simulink model "comboPlusKirschBinarized"  (R2024a)
settings: Solver=FixedStepDiscrete  StartTime=0.0  StopTime=1  RelTol=1e-3
undefined symbols (not defined in the file or in its folder): dx, dy, G, KirschThrL, KirschThrS, MagThr, north, northWest, southWest, west
libraries: visionsinks x10, hdlsllib x8, visionsources x1
Description:
  | Sobel Edge Detection Using the MATLAB(R) Function Block
  | This example shows how to use HDL Coder(TM) to check,
  | generate, and verify HDL code for a Sobel Edge Detection
  | block built using the MATLAB Function block.
settings Model: FPTRunName=Active  Creator=The MathWorks, Inc.  LastModifiedBy=dskap
settings SolverCC: AlgebraicLoopSolver=TrustRegion
settings DataIOCC: LimitDataPoints=on  SaveFormat=Array  SignalLogging=off  ReturnWorkspaceOutputs=off
settings OptimizationCC: BlockReduction=off  ConditionallyExecuteInputs=off  DefaultParameterBehavior=Inlined  ExpressionDepthLimit=2147483647  InitFltsAndDblsToZero=on  EfficientMapNaN2IntZero=off  LifeSpan=inf
settings DebuggingCC: AlgebraicLoopMsg=error  SaveWithParameterizedLinksMsg=none  UnderspecifiedInitializationDetection=Classic  MergeDetectMultiDrivingBlocksExec=none  SignalResolutionControl=TryResolveAllWithWarning  MultiTaskDSMMsg=warning  MultiTaskCondExecSysMsg=none  SingleTaskRateTransMsg=error  IntegerOverflowMsg=none  ParameterPrecisionLossMsg=none  FcnCallInpInsideContextMsg=warning  UnconnectedInputMsg=warning  UnconnectedOutputMsg=warning  UnconnectedLineMsg=warning  AllowSymbolicDim=off  StateNameClashWarn=warning  StrictBusMsg=ErrorOnBusTreatedAsVector  SFUnexpectedBacktrackingDiag=warning  SFNoUnconditionalDefaultTransitionDiag=warning  SFExecutionAtInitializationDiag=none  IntegerSaturationMsg=none  ArithmeticOperatorsInVariantConditions=warning
settings HardwareCC: ProdBitPerPointer=32  ProdBitPerSizeT=32  ProdBitPerPtrDiffT=32  ProdLargestAtomicFloat=None  ProdIntDivRoundTo=Undefined  ProdEndianess=Unspecified  ProdWordSize=32  ProdHWDeviceType=ASIC/FPGA  TargetHWDeviceType=32-bit Generic  ProdEqTarget=off
settings ModelReferenceCC: EnableRefExpFcnMdlSchedulingChecks=on  PropagateSignalLabelsOutOfModel=off
settings SFSimCC: SimUseLocalCustomCode=off  CustomCodeUndefinedFunction=UseInterfaceOnly
settings RTWCC: RTWUseLocalCustomCode=off  GPUComputeCapability=3.5  DLArmComputeVersion=19.05
settings CodeAppCC: StateflowObjectComments=on
settings GRTTargetCC: TargetFcnLib=ansi_tfl_tmw.mat  TargetLangStandard=C89/C90 (ANSI)  CombineOutputUpdateFcns=off  GRTInterface=on
settings ConfigComp: CovMetricSettings=dw  CovSaveCumulativeToWorkspaceVar=on  CovSaveSingleToWorkspaceVar=on  CovExternalEMLEnable=off

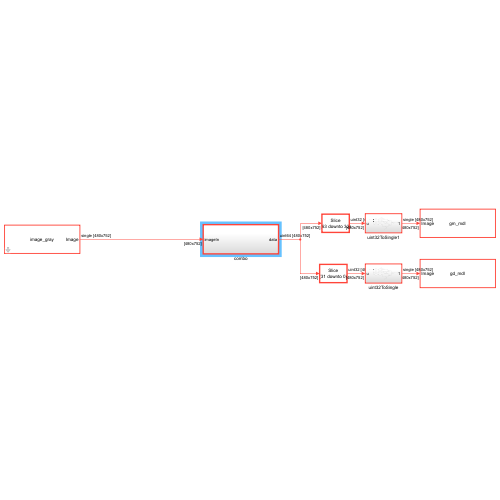
[thumbnail: Simulink's stored preview of the top-level diagram]
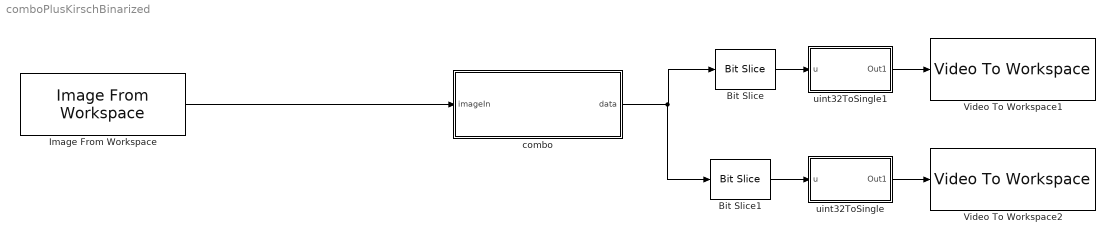
== system comboPlusKirschBinarized ==
  Bit Slice : hdlsllib/Logic and Bit Operations/Bit Slice  lidx=63  ridx=32
  Bit Slice1 : hdlsllib/Logic and Bit Operations/Bit Slice  lidx=31  ridx=0
  Image From Workspace : visionsources/Image From Workspace  Tag=vipblks_nd  ImageValue=image_gray  Ts=1  imagePorts=One multidimensional signal  OutPortLabels=R|G|B  ImageDataType=Inherit from 'Value'  Signed=on  WordLength=16  sdImageDataType=sfix(16)  FractionLengthMode=User-defined  FractionLength=15
  Video To Workspace1 : visionsinks/Video To Workspace  VariableName=gm_mdl  NumInputs=1  DataLimit=1  DecimationFactor=1  LogFi=off  InPortLabels=R|G|B
  Video To Workspace2 : visionsinks/Video To Workspace  VariableName=gd_mdl  NumInputs=1  DataLimit=1  DecimationFactor=1  LogFi=off  InPortLabels=R|G|B
  combo : Subsystem  TreatAsAtomicUnit=on
  uint32ToSingle : Subsystem
  uint32ToSingle1 : Subsystem
  wires:
  Image From Workspace/1 -> combo/1(imageIn)
  combo/1(data) -> Bit Slice1/1, Bit Slice/1
  Bit Slice/1 -> uint32ToSingle1/1(u)
  uint32ToSingle1/1(Out1) -> Video To Workspace1/1
  uint32ToSingle/1(Out1) -> Video To Workspace2/1
  Bit Slice1/1 -> uint32ToSingle/1(u)

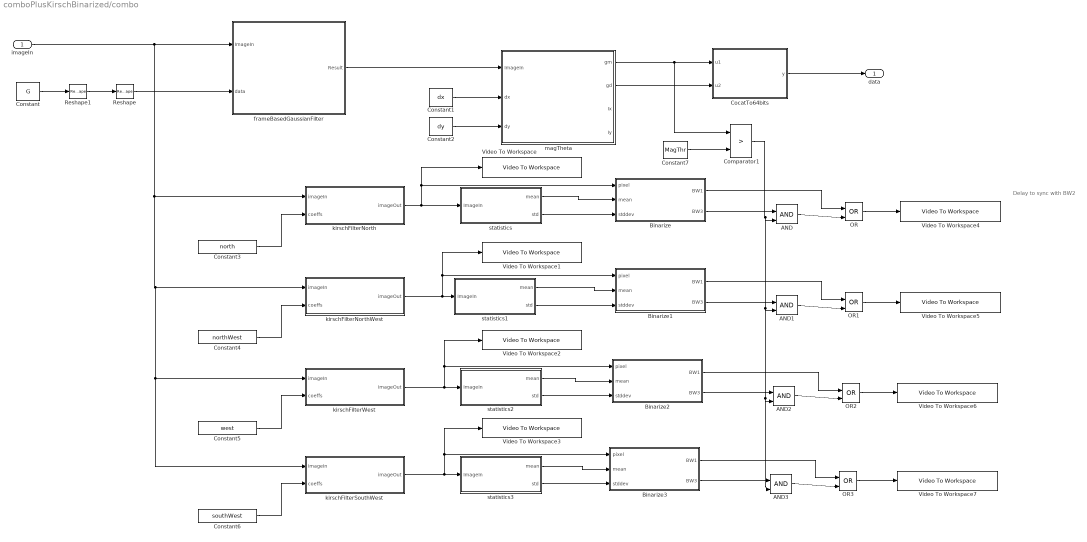
== system comboPlusKirschBinarized/combo ==
  note: Delay to sync with BW2
  imageIn : Inport
  AND{,1..3} (4 alike) : Logic  IconShape=distinctive  AllPortsSameDT=off  OutDataTypeStr=boolean
  Binarize : Subsystem
  Binarize1 : Subsystem
  Binarize2 : Subsystem
  Binarize3 : Subsystem
  CocatTo64bits : MATLAB Function  TreatAsAtomicUnit=on
  Comparator1 : RelationalOperator  Operator=>  OutDataTypeStr=boolean  RndMeth=Simplest  InputSameDT=off
  Constant : Constant  Value=G  OutDataTypeStr=single  SampleTime=-1
  Constant1 : Constant  Value=dx  SampleTime=-1
  Constant2 : Constant  Value=dy  SampleTime=-1
  Constant3 : Constant  Value=north  SampleTime=-1
  Constant4 : Constant  Value=northWest  SampleTime=-1
  Constant5 : Constant  Value=west  SampleTime=-1
  Constant6 : Constant  Value=southWest  SampleTime=-1
  Constant7 : Constant  Value=MagThr  SampleTime=-1
  OR{,1..3} (4 alike) : Logic  Operator=OR  IconShape=distinctive  AllPortsSameDT=off  OutDataTypeStr=boolean
  Reshape : Reshape  OutputDimensionality=Customize  OutputDimensions=[3,3]
  Reshape1 : Reshape
  Video To Workspace : visionsinks/Video To Workspace  VariableName=dirMagNorth_mdl  NumInputs=1  DataLimit=1  DecimationFactor=1  LogFi=off  InPortLabels=R|G|B
  Video To Workspace1 : visionsinks/Video To Workspace  VariableName=dirMagNorthWest_mdl  NumInputs=1  DataLimit=1  DecimationFactor=1  LogFi=off  InPortLabels=R|G|B
  Video To Workspace2 : visionsinks/Video To Workspace  VariableName=dirMagWest_mdl  NumInputs=1  DataLimit=1  DecimationFactor=1  LogFi=off  InPortLabels=R|G|B
  Video To Workspace3 : visionsinks/Video To Workspace  VariableName=dirMagSouthWest_mdl  NumInputs=1  DataLimit=1  DecimationFactor=1  LogFi=off  InPortLabels=R|G|B
  Video To Workspace4 : visionsinks/Video To Workspace  VariableName=dirMagNorthBW_mdl  NumInputs=1  DataLimit=1  DecimationFactor=1  LogFi=off  InPortLabels=R|G|B
  Video To Workspace5 : visionsinks/Video To Workspace  VariableName=dirMagNorthWestBW_mdl  NumInputs=1  DataLimit=1  DecimationFactor=1  LogFi=off  InPortLabels=R|G|B
  Video To Workspace6 : visionsinks/Video To Workspace  VariableName=dirMagWestBW_mdl  NumInputs=1  DataLimit=1  DecimationFactor=1  LogFi=off  InPortLabels=R|G|B
  Video To Workspace7 : visionsinks/Video To Workspace  VariableName=dirMagSouthWestBW_mdl  NumInputs=1  DataLimit=1  DecimationFactor=1  LogFi=off  InPortLabels=R|G|B
  frameBasedGaussianFilter : MATLAB Function  TreatAsAtomicUnit=on
  kirschFilterNorth : Subsystem  TreatAsAtomicUnit=on
  kirschFilterNorthWest : Subsystem  TreatAsAtomicUnit=on
  kirschFilterSouthWest : Subsystem  TreatAsAtomicUnit=on
  kirschFilterWest : Subsystem  TreatAsAtomicUnit=on
  magTheta : MATLAB Function  TreatAsAtomicUnit=on
  statistics : Subsystem
  statistics1 : Subsystem
  statistics2 : Subsystem
  statistics3 : Subsystem
  data : Outport
  wires:
  Reshape1/1 -> Reshape/1
  frameBasedGaussianFilter/1(Result) -> magTheta/1(ImageIn)
  Reshape/1 -> frameBasedGaussianFilter/2(data)
  Constant/1 -> Reshape1/1
  Constant1/1 -> magTheta/2(dx)
  Constant2/1 -> magTheta/3(dy)
  magTheta/1(gm) -> Comparator1/1, CocatTo64bits/1(u1)
  magTheta/2(gd) -> CocatTo64bits/2(u2)
  CocatTo64bits/1(y) -> data/1
  Constant6/1 -> kirschFilterSouthWest/2(coeffs)
  kirschFilterWest/1(imageOut) -> statistics2/1(ImageIn), Video To Workspace2/1, Binarize2/1(pixel)
  Constant4/1 -> kirschFilterNorthWest/2(coeffs)
  kirschFilterSouthWest/1(imageOut) -> statistics3/1(ImageIn), Video To Workspace3/1, Binarize3/1(pixel)
  kirschFilterNorth/1(imageOut) -> Video To Workspace/1, Binarize/1(pixel), statistics/1(ImageIn)
  imageIn/1 -> kirschFilterSouthWest/1(imageIn), kirschFilterWest/1(imageIn), kirschFilterNorthWest/1(imageIn), kirschFilterNorth/1(imageIn), frameBasedGaussianFilter/1(ImageIn)
  Constant5/1 -> kirschFilterWest/2(coeffs)
  kirschFilterNorthWest/1(imageOut) -> statistics1/1(ImageIn), Video To Workspace1/1, Binarize1/1(pixel)
  Constant3/1 -> kirschFilterNorth/2(coeffs)
  Constant7/1 -> Comparator1/2
  statistics/1(mean) -> Binarize/2(mean)
  statistics/2(std) -> Binarize/3(stddev)
  statistics1/2(std) -> Binarize1/3(stddev)
  statistics1/1(mean) -> Binarize1/2(mean)
  statistics2/1(mean) -> Binarize2/2(mean)
  statistics2/2(std) -> Binarize2/3(stddev)
  statistics3/1(mean) -> Binarize3/2(mean)
  statistics3/2(std) -> Binarize3/3(stddev)
  Binarize/1(BW1) -> OR/1
  Binarize/2(BW3) -> AND/1
  AND/1 -> OR/2
  OR/1 -> Video To Workspace4/1
  Binarize1/1(BW1) -> OR1/1
  OR1/1 -> Video To Workspace5/1
  Binarize1/2(BW3) -> AND1/1
  AND1/1 -> OR1/2
  Binarize2/1(BW1) -> OR2/1
  OR2/1 -> Video To Workspace6/1
  Binarize2/2(BW3) -> AND2/1
  AND2/1 -> OR2/2
  Comparator1/1 -> AND3/2, AND2/2, AND1/2, AND/2
  Binarize3/1(BW1) -> OR3/1
  OR3/1 -> Video To Workspace7/1
  Binarize3/2(BW3) -> AND3/1
  AND3/1 -> OR3/2

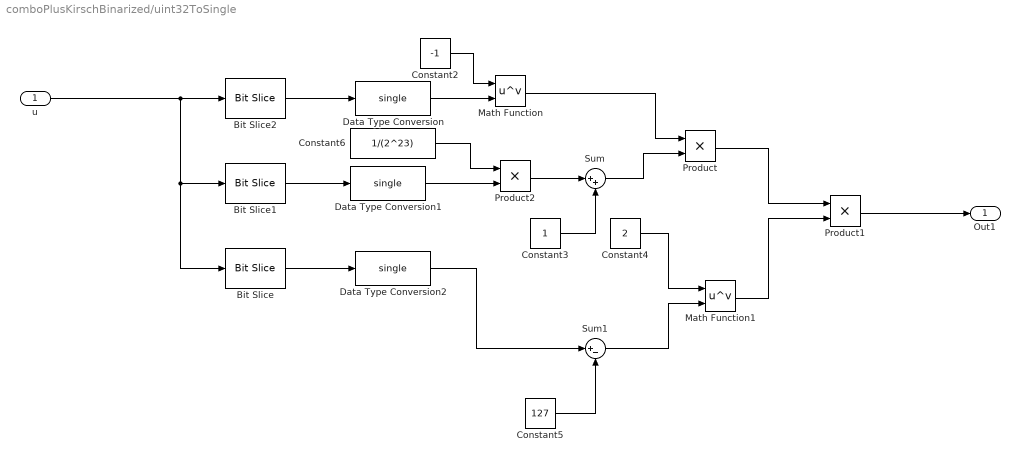
== system comboPlusKirschBinarized/uint32ToSingle ==
  u : Inport
  Bit Slice : hdlsllib/Logic and Bit Operations/Bit Slice  lidx=30  ridx=23
  Bit Slice1 : hdlsllib/Logic and Bit Operations/Bit Slice  lidx=22  ridx=0
  Bit Slice2 : hdlsllib/Logic and Bit Operations/Bit Slice  lidx=31  ridx=31
  Constant2 : Constant  Value=-1  OutDataTypeStr=single  SampleTime=-1
  Constant3 : Constant  OutDataTypeStr=single  SampleTime=-1
  Constant4 : Constant  Value=2  OutDataTypeStr=single  SampleTime=-1
  Constant5 : Constant  Value=127  OutDataTypeStr=single  SampleTime=-1
  Constant6 : Constant  Value=1/(2^23)  OutDataTypeStr=single  SampleTime=-1
  Data Type Conversion : DataTypeConversion  OutDataTypeStr=single  SaturateOnIntegerOverflow=off  RndMeth=Floor
  Data Type Conversion1 : DataTypeConversion  OutDataTypeStr=single  SaturateOnIntegerOverflow=off  RndMeth=Floor
  Data Type Conversion2 : DataTypeConversion  OutDataTypeStr=single  SaturateOnIntegerOverflow=off  RndMeth=Floor
  Math Function : Math  Operator=pow
  Math Function1 : Math  Operator=pow
  Product : Product
  Product1 : Product
  Product2 : Product
  Sum : Sum  Inputs=|++
  Sum1 : Sum  Inputs=|+-
  Out1 : Outport
  wires:
  Product1/1 -> Out1/1
  Bit Slice1/1 -> Data Type Conversion1/1
  Data Type Conversion/1 -> Math Function/2
  Math Function1/1 -> Product1/2
  u/1 -> Bit Slice1/1, Bit Slice/1, Bit Slice2/1
  Constant4/1 -> Math Function1/1
  Product2/1 -> Sum/1
  Bit Slice2/1 -> Data Type Conversion/1
  Sum1/1 -> Math Function1/2
  Constant5/1 -> Sum1/2
  Math Function/1 -> Product/1
  Bit Slice/1 -> Data Type Conversion2/1
  Constant2/1 -> Math Function/1
  Sum/1 -> Product/2
  Product/1 -> Product1/1
  Data Type Conversion1/1 -> Product2/2
  Constant3/1 -> Sum/2
  Data Type Conversion2/1 -> Sum1/1
  Constant6/1 -> Product2/1

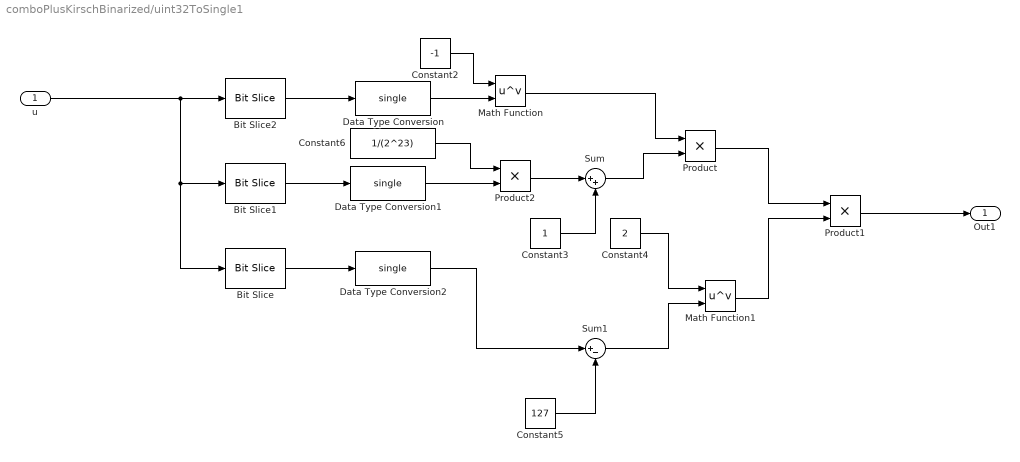
== system comboPlusKirschBinarized/uint32ToSingle1 ==
  u : Inport
  Bit Slice : hdlsllib/Logic and Bit Operations/Bit Slice  lidx=30  ridx=23
  Bit Slice1 : hdlsllib/Logic and Bit Operations/Bit Slice  lidx=22  ridx=0
  Bit Slice2 : hdlsllib/Logic and Bit Operations/Bit Slice  lidx=31  ridx=31
  Constant2 : Constant  Value=-1  OutDataTypeStr=single  SampleTime=-1
  Constant3 : Constant  OutDataTypeStr=single  SampleTime=-1
  Constant4 : Constant  Value=2  OutDataTypeStr=single  SampleTime=-1
  Constant5 : Constant  Value=127  OutDataTypeStr=single  SampleTime=-1
  Constant6 : Constant  Value=1/(2^23)  OutDataTypeStr=single  SampleTime=-1
  Data Type Conversion : DataTypeConversion  OutDataTypeStr=single  SaturateOnIntegerOverflow=off  RndMeth=Floor
  Data Type Conversion1 : DataTypeConversion  OutDataTypeStr=single  SaturateOnIntegerOverflow=off  RndMeth=Floor
  Data Type Conversion2 : DataTypeConversion  OutDataTypeStr=single  SaturateOnIntegerOverflow=off  RndMeth=Floor
  Math Function : Math  Operator=pow
  Math Function1 : Math  Operator=pow
  Product : Product
  Product1 : Product
  Product2 : Product
  Sum : Sum  Inputs=|++
  Sum1 : Sum  Inputs=|+-
  Out1 : Outport
  wires:
  Constant6/1 -> Product2/1
  Data Type Conversion2/1 -> Sum1/1
  Constant3/1 -> Sum/2
  Data Type Conversion1/1 -> Product2/2
  Product/1 -> Product1/1
  Sum/1 -> Product/2
  Constant2/1 -> Math Function/1
  Bit Slice/1 -> Data Type Conversion2/1
  Math Function/1 -> Product/1
  Constant5/1 -> Sum1/2
  Sum1/1 -> Math Function1/2
  Bit Slice2/1 -> Data Type Conversion/1
  Product2/1 -> Sum/1
  Constant4/1 -> Math Function1/1
  u/1 -> Bit Slice2/1, Bit Slice/1, Bit Slice1/1
  Math Function1/1 -> Product1/2
  Data Type Conversion/1 -> Math Function/2
  Bit Slice1/1 -> Data Type Conversion1/1
  Product1/1 -> Out1/1

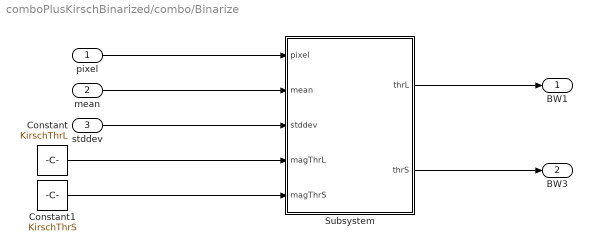
== system comboPlusKirschBinarized/combo/Binarize ==
  pixel : Inport
  mean : Inport  Port=2
  stddev : Inport  Port=3
  Constant : Constant  Value=KirschThrL  SampleTime=-1
  Constant1 : Constant  Value=KirschThrS  SampleTime=-1
  Subsystem : Subsystem
  BW1 : Outport
  BW3 : Outport  Port=2
  wires:
  pixel/1 -> Subsystem/1(pixel)
  mean/1 -> Subsystem/2(mean)
  stddev/1 -> Subsystem/3(stddev)
  Subsystem/1(thrL) -> BW1/1
  Subsystem/2(thrS) -> BW3/1
  Constant/1 -> Subsystem/4(magThrL)
  Constant1/1 -> Subsystem/5(magThrS)

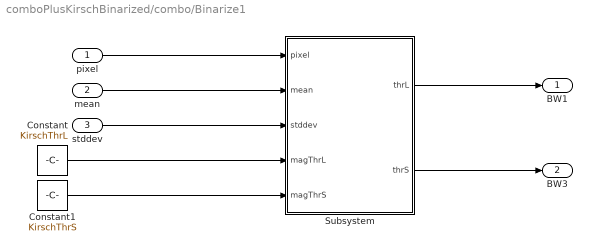
== system comboPlusKirschBinarized/combo/Binarize1 ==
  pixel : Inport
  mean : Inport  Port=2
  stddev : Inport  Port=3
  Constant : Constant  Value=KirschThrL  SampleTime=-1
  Constant1 : Constant  Value=KirschThrS  SampleTime=-1
  Subsystem : Subsystem
  BW1 : Outport
  BW3 : Outport  Port=2
  wires:
  pixel/1 -> Subsystem/1(pixel)
  mean/1 -> Subsystem/2(mean)
  stddev/1 -> Subsystem/3(stddev)
  Subsystem/1(thrL) -> BW1/1
  Subsystem/2(thrS) -> BW3/1
  Constant/1 -> Subsystem/4(magThrL)
  Constant1/1 -> Subsystem/5(magThrS)

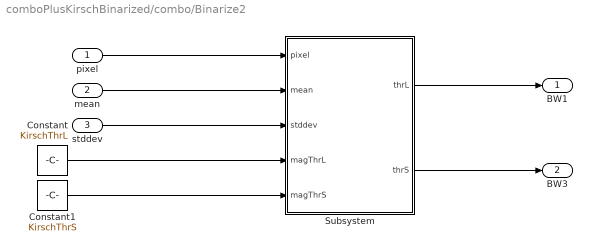
== system comboPlusKirschBinarized/combo/Binarize2 ==
  pixel : Inport
  mean : Inport  Port=2
  stddev : Inport  Port=3
  Constant : Constant  Value=KirschThrL  SampleTime=-1
  Constant1 : Constant  Value=KirschThrS  SampleTime=-1
  Subsystem : Subsystem
  BW1 : Outport
  BW3 : Outport  Port=2
  wires:
  pixel/1 -> Subsystem/1(pixel)
  mean/1 -> Subsystem/2(mean)
  stddev/1 -> Subsystem/3(stddev)
  Subsystem/1(thrL) -> BW1/1
  Subsystem/2(thrS) -> BW3/1
  Constant/1 -> Subsystem/4(magThrL)
  Constant1/1 -> Subsystem/5(magThrS)

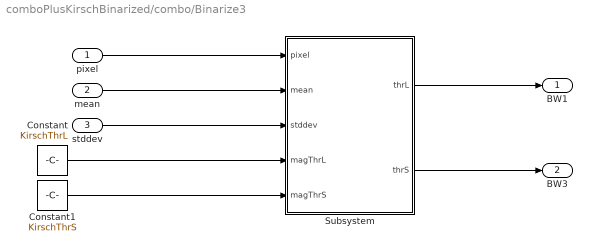
== system comboPlusKirschBinarized/combo/Binarize3 ==
  pixel : Inport
  mean : Inport  Port=2
  stddev : Inport  Port=3
  Constant : Constant  Value=KirschThrL  SampleTime=-1
  Constant1 : Constant  Value=KirschThrS  SampleTime=-1
  Subsystem : Subsystem
  BW1 : Outport
  BW3 : Outport  Port=2
  wires:
  pixel/1 -> Subsystem/1(pixel)
  mean/1 -> Subsystem/2(mean)
  stddev/1 -> Subsystem/3(stddev)
  Subsystem/1(thrL) -> BW1/1
  Subsystem/2(thrS) -> BW3/1
  Constant/1 -> Subsystem/4(magThrL)
  Constant1/1 -> Subsystem/5(magThrS)

== system comboPlusKirschBinarized/combo/kirschFilterNorth ==
  imageIn : Inport
  coeffs : Inport  Port=2
  frameBasedKirschFilter : MATLAB Function  TreatAsAtomicUnit=on
  imageOut : Outport
  wires:
  imageIn/1 -> frameBasedKirschFilter/1(ImageIn)
  frameBasedKirschFilter/1(Result) -> imageOut/1
  coeffs/1 -> frameBasedKirschFilter/2(data)

== system comboPlusKirschBinarized/combo/kirschFilterNorthWest ==
  imageIn : Inport
  coeffs : Inport  Port=2
  frameBasedKirschFilter : MATLAB Function  TreatAsAtomicUnit=on
  imageOut : Outport
  wires:
  imageIn/1 -> frameBasedKirschFilter/1(ImageIn)
  frameBasedKirschFilter/1(Result) -> imageOut/1
  coeffs/1 -> frameBasedKirschFilter/2(data)

== system comboPlusKirschBinarized/combo/kirschFilterSouthWest ==
  imageIn : Inport
  coeffs : Inport  Port=2
  frameBasedKirschFilter : MATLAB Function  TreatAsAtomicUnit=on
  imageOut : Outport
  wires:
  imageIn/1 -> frameBasedKirschFilter/1(ImageIn)
  frameBasedKirschFilter/1(Result) -> imageOut/1
  coeffs/1 -> frameBasedKirschFilter/2(data)

== system comboPlusKirschBinarized/combo/kirschFilterWest ==
  imageIn : Inport
  coeffs : Inport  Port=2
  frameBasedKirschFilter : MATLAB Function  TreatAsAtomicUnit=on
  imageOut : Outport
  wires:
  imageIn/1 -> frameBasedKirschFilter/1(ImageIn)
  frameBasedKirschFilter/1(Result) -> imageOut/1
  coeffs/1 -> frameBasedKirschFilter/2(data)

== system comboPlusKirschBinarized/combo/statistics ==
  ImageIn : Inport
  frameBasedMean : MATLAB Function  TreatAsAtomicUnit=on
  frameBasedStd : MATLAB Function  TreatAsAtomicUnit=on
  mean : Outport
  std : Outport  Port=2
  wires:
  frameBasedMean/1(Result) -> mean/1, frameBasedStd/2(mean)
  frameBasedStd/1(Result) -> std/1
  ImageIn/1 -> frameBasedStd/1(ImageIn), frameBasedMean/1(ImageIn)

== system comboPlusKirschBinarized/combo/statistics1 ==
  ImageIn : Inport
  frameBasedMean : MATLAB Function  TreatAsAtomicUnit=on
  frameBasedStd : MATLAB Function  TreatAsAtomicUnit=on
  mean : Outport
  std : Outport  Port=2
  wires:
  ImageIn/1 -> frameBasedMean/1(ImageIn), frameBasedStd/1(ImageIn)
  frameBasedStd/1(Result) -> std/1
  frameBasedMean/1(Result) -> frameBasedStd/2(mean), mean/1

== system comboPlusKirschBinarized/combo/statistics2 ==
  ImageIn : Inport
  frameBasedMean : MATLAB Function  TreatAsAtomicUnit=on
  frameBasedStd : MATLAB Function  TreatAsAtomicUnit=on
  mean : Outport
  std : Outport  Port=2
  wires:
  frameBasedMean/1(Result) -> mean/1, frameBasedStd/2(mean)
  frameBasedStd/1(Result) -> std/1
  ImageIn/1 -> frameBasedStd/1(ImageIn), frameBasedMean/1(ImageIn)

== system comboPlusKirschBinarized/combo/statistics3 ==
  ImageIn : Inport
  frameBasedMean : MATLAB Function  TreatAsAtomicUnit=on
  frameBasedStd : MATLAB Function  TreatAsAtomicUnit=on
  mean : Outport
  std : Outport  Port=2
  wires:
  ImageIn/1 -> frameBasedMean/1(ImageIn), frameBasedStd/1(ImageIn)
  frameBasedStd/1(Result) -> std/1
  frameBasedMean/1(Result) -> frameBasedStd/2(mean), mean/1

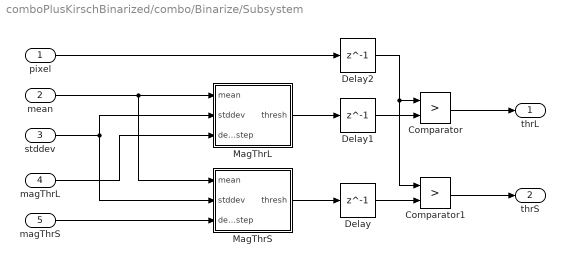
== system comboPlusKirschBinarized/combo/Binarize/Subsystem ==
  pixel : Inport
  mean : Inport  Port=2
  stddev : Inport  Port=3
  magThrL : Inport  Port=4
  magThrS : Inport  Port=5
  Comparator : RelationalOperator  Operator=>  OutDataTypeStr=boolean  RndMeth=Simplest  InputSameDT=off
  Comparator1 : RelationalOperator  Operator=>  OutDataTypeStr=boolean  RndMeth=Simplest  InputSameDT=off
  Delay : Delay  DelayLength=1
  Delay1 : Delay  DelayLength=1
  Delay2 : Delay  DelayLength=1
  MagThrL : Subsystem
  MagThrS : Subsystem
  thrL : Outport  InitialOutput=0
  thrS : Outport  Port=2  InitialOutput=0
  wires:
  pixel/1 -> Delay2/1
  MagThrL/1(thresh) -> Delay1/1
  magThrS/1 -> MagThrS/3(dev_step)
  MagThrS/1(thresh) -> Delay/1
  magThrL/1 -> MagThrL/3(dev_step)
  mean/1 -> MagThrS/1(mean), MagThrL/1(mean)
  stddev/1 -> MagThrS/2(stddev), MagThrL/2(stddev)
  Comparator1/1 -> thrS/1
  Comparator/1 -> thrL/1
  Delay/1 -> Comparator1/2
  Delay1/1 -> Comparator/2
  Delay2/1 -> Comparator1/1, Comparator/1

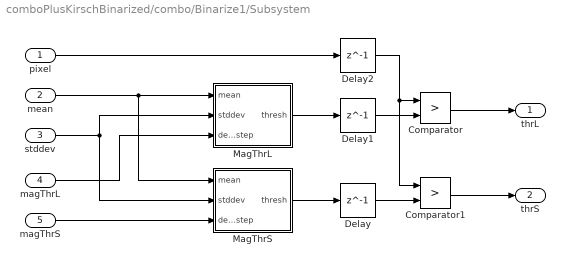
== system comboPlusKirschBinarized/combo/Binarize1/Subsystem ==
  pixel : Inport
  mean : Inport  Port=2
  stddev : Inport  Port=3
  magThrL : Inport  Port=4
  magThrS : Inport  Port=5
  Comparator : RelationalOperator  Operator=>  OutDataTypeStr=boolean  RndMeth=Simplest  InputSameDT=off
  Comparator1 : RelationalOperator  Operator=>  OutDataTypeStr=boolean  RndMeth=Simplest  InputSameDT=off
  Delay : Delay  DelayLength=1
  Delay1 : Delay  DelayLength=1
  Delay2 : Delay  DelayLength=1
  MagThrL : Subsystem
  MagThrS : Subsystem
  thrL : Outport  InitialOutput=0
  thrS : Outport  Port=2  InitialOutput=0
  wires:
  pixel/1 -> Delay2/1
  MagThrL/1(thresh) -> Delay1/1
  magThrS/1 -> MagThrS/3(dev_step)
  MagThrS/1(thresh) -> Delay/1
  magThrL/1 -> MagThrL/3(dev_step)
  mean/1 -> MagThrS/1(mean), MagThrL/1(mean)
  stddev/1 -> MagThrS/2(stddev), MagThrL/2(stddev)
  Comparator1/1 -> thrS/1
  Comparator/1 -> thrL/1
  Delay/1 -> Comparator1/2
  Delay1/1 -> Comparator/2
  Delay2/1 -> Comparator1/1, Comparator/1

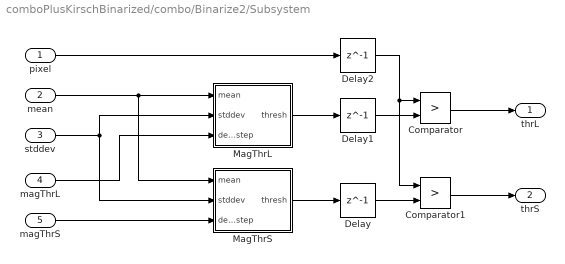
== system comboPlusKirschBinarized/combo/Binarize2/Subsystem ==
  pixel : Inport
  mean : Inport  Port=2
  stddev : Inport  Port=3
  magThrL : Inport  Port=4
  magThrS : Inport  Port=5
  Comparator : RelationalOperator  Operator=>  OutDataTypeStr=boolean  RndMeth=Simplest  InputSameDT=off
  Comparator1 : RelationalOperator  Operator=>  OutDataTypeStr=boolean  RndMeth=Simplest  InputSameDT=off
  Delay : Delay  DelayLength=1
  Delay1 : Delay  DelayLength=1
  Delay2 : Delay  DelayLength=1
  MagThrL : Subsystem
  MagThrS : Subsystem
  thrL : Outport  InitialOutput=0
  thrS : Outport  Port=2  InitialOutput=0
  wires:
  pixel/1 -> Delay2/1
  MagThrL/1(thresh) -> Delay1/1
  magThrS/1 -> MagThrS/3(dev_step)
  MagThrS/1(thresh) -> Delay/1
  magThrL/1 -> MagThrL/3(dev_step)
  mean/1 -> MagThrS/1(mean), MagThrL/1(mean)
  stddev/1 -> MagThrS/2(stddev), MagThrL/2(stddev)
  Comparator1/1 -> thrS/1
  Comparator/1 -> thrL/1
  Delay/1 -> Comparator1/2
  Delay1/1 -> Comparator/2
  Delay2/1 -> Comparator1/1, Comparator/1

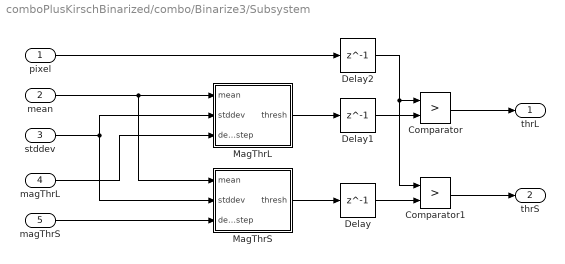
== system comboPlusKirschBinarized/combo/Binarize3/Subsystem ==
  pixel : Inport
  mean : Inport  Port=2
  stddev : Inport  Port=3
  magThrL : Inport  Port=4
  magThrS : Inport  Port=5
  Comparator : RelationalOperator  Operator=>  OutDataTypeStr=boolean  RndMeth=Simplest  InputSameDT=off
  Comparator1 : RelationalOperator  Operator=>  OutDataTypeStr=boolean  RndMeth=Simplest  InputSameDT=off
  Delay : Delay  DelayLength=1
  Delay1 : Delay  DelayLength=1
  Delay2 : Delay  DelayLength=1
  MagThrL : Subsystem
  MagThrS : Subsystem
  thrL : Outport  InitialOutput=0
  thrS : Outport  Port=2  InitialOutput=0
  wires:
  pixel/1 -> Delay2/1
  MagThrL/1(thresh) -> Delay1/1
  magThrS/1 -> MagThrS/3(dev_step)
  MagThrS/1(thresh) -> Delay/1
  magThrL/1 -> MagThrL/3(dev_step)
  mean/1 -> MagThrS/1(mean), MagThrL/1(mean)
  stddev/1 -> MagThrS/2(stddev), MagThrL/2(stddev)
  Comparator1/1 -> thrS/1
  Comparator/1 -> thrL/1
  Delay/1 -> Comparator1/2
  Delay1/1 -> Comparator/2
  Delay2/1 -> Comparator1/1, Comparator/1

== system comboPlusKirschBinarized/combo/Binarize/Subsystem/MagThrL ==
  mean : Inport
  stddev : Inport  Port=2
  dev_step : Inport  Port=3
  Add1 : Sum
  Product : Product
  thresh : Outport
  wires:
  stddev/1 -> Product/1
  mean/1 -> Add1/1
  dev_step/1 -> Product/2
  Product/1 -> Add1/2
  Add1/1 -> thresh/1

== system comboPlusKirschBinarized/combo/Binarize/Subsystem/MagThrS ==
  mean : Inport
  stddev : Inport  Port=2
  dev_step : Inport  Port=3
  Add1 : Sum
  Product : Product
  thresh : Outport
  wires:
  stddev/1 -> Product/1
  mean/1 -> Add1/1
  dev_step/1 -> Product/2
  Product/1 -> Add1/2
  Add1/1 -> thresh/1

== system comboPlusKirschBinarized/combo/Binarize1/Subsystem/MagThrL ==
  mean : Inport
  stddev : Inport  Port=2
  dev_step : Inport  Port=3
  Add1 : Sum
  Product : Product
  thresh : Outport
  wires:
  stddev/1 -> Product/1
  mean/1 -> Add1/1
  dev_step/1 -> Product/2
  Product/1 -> Add1/2
  Add1/1 -> thresh/1

== system comboPlusKirschBinarized/combo/Binarize1/Subsystem/MagThrS ==
  mean : Inport
  stddev : Inport  Port=2
  dev_step : Inport  Port=3
  Add1 : Sum
  Product : Product
  thresh : Outport
  wires:
  stddev/1 -> Product/1
  mean/1 -> Add1/1
  dev_step/1 -> Product/2
  Product/1 -> Add1/2
  Add1/1 -> thresh/1

== system comboPlusKirschBinarized/combo/Binarize2/Subsystem/MagThrL ==
  mean : Inport
  stddev : Inport  Port=2
  dev_step : Inport  Port=3
  Add1 : Sum
  Product : Product
  thresh : Outport
  wires:
  stddev/1 -> Product/1
  mean/1 -> Add1/1
  dev_step/1 -> Product/2
  Product/1 -> Add1/2
  Add1/1 -> thresh/1

== system comboPlusKirschBinarized/combo/Binarize2/Subsystem/MagThrS ==
  mean : Inport
  stddev : Inport  Port=2
  dev_step : Inport  Port=3
  Add1 : Sum
  Product : Product
  thresh : Outport
  wires:
  stddev/1 -> Product/1
  mean/1 -> Add1/1
  dev_step/1 -> Product/2
  Product/1 -> Add1/2
  Add1/1 -> thresh/1

== system comboPlusKirschBinarized/combo/Binarize3/Subsystem/MagThrL ==
  mean : Inport
  stddev : Inport  Port=2
  dev_step : Inport  Port=3
  Add1 : Sum
  Product : Product
  thresh : Outport
  wires:
  stddev/1 -> Product/1
  mean/1 -> Add1/1
  dev_step/1 -> Product/2
  Product/1 -> Add1/2
  Add1/1 -> thresh/1

== system comboPlusKirschBinarized/combo/Binarize3/Subsystem/MagThrS ==
  mean : Inport
  stddev : Inport  Port=2
  dev_step : Inport  Port=3
  Add1 : Sum
  Product : Product
  thresh : Outport
  wires:
  stddev/1 -> Product/1
  mean/1 -> Add1/1
  dev_step/1 -> Product/2
  Product/1 -> Add1/2
  Add1/1 -> thresh/1

== matlab function comboPlusKirschBinarized/combo/statistics1/frameBasedStd ==
  data: Result output; ImageIn input; mean input
function Result   = frameBasedStd(ImageIn, mean)
    accumulator2 = single(0);
    Result = hdl.iteratorfun(@max_fun2, ImageIn, accumulator2,mean); 
end
 
function accumulator2 = max_fun2(sample, accumulator2, idx, mean)
    numPix = 40000;  
    temp = (sample-mean)^2;
  accumulator2 = accumulator2 + temp;
  
  if idx == numPix
    accumulator2 = (accumulator2/(numPix - 1))^.5;
  end
end

== matlab function comboPlusKirschBinarized/combo/statistics2/frameBasedMean ==
  data: Result output; ImageIn input
function Result   = frameBasedMean(ImageIn)
    accumulator = single(0);    
    Result = hdl.iteratorfun(@max_fun, ImageIn, accumulator);
end
 
function accumulator = max_fun(sample, accumulator, idx)
  numPix = 40000;
  accumulator = accumulator + sample;
  if idx == numPix
    accumulator = single(accumulator / numPix);
  end
end

== matlab function comboPlusKirschBinarized/combo/statistics2/frameBasedStd ==
  data: Result output; ImageIn input; mean input
function Result   = frameBasedStd(ImageIn, mean)
    accumulator2 = single(0);
    Result = hdl.iteratorfun(@max_fun2, ImageIn, accumulator2,mean); 
end
 
function accumulator2 = max_fun2(sample, accumulator2, idx, mean)
    numPix = 40000;  
    temp = (sample-mean)^2;
  accumulator2 = accumulator2 + temp;
  
  if idx == numPix
    accumulator2 = (accumulator2/(numPix - 1))^.5;
  end
end

== matlab function comboPlusKirschBinarized/combo/statistics3/frameBasedMean ==
  data: Result output; ImageIn input
function Result   = frameBasedMean(ImageIn)
    accumulator = single(0);    
    Result = hdl.iteratorfun(@max_fun, ImageIn, accumulator);
end
 
function accumulator = max_fun(sample, accumulator, idx)
  numPix = 40000;
  accumulator = accumulator + sample;
  if idx == numPix
    accumulator = single(accumulator / numPix);
  end
end

== matlab function comboPlusKirschBinarized/combo/statistics3/frameBasedStd ==
  data: Result output; ImageIn input; mean input
function Result   = frameBasedStd(ImageIn, mean)
    accumulator2 = single(0);
    Result = hdl.iteratorfun(@max_fun2, ImageIn, accumulator2,mean); 
end
 
function accumulator2 = max_fun2(sample, accumulator2, idx, mean)
    numPix = 40000;  
    temp = (sample-mean)^2;
  accumulator2 = accumulator2 + temp;
  
  if idx == numPix
    accumulator2 = (accumulator2/(numPix - 1))^.5;
  end
end

== matlab function comboPlusKirschBinarized/combo/magTheta ==
  data: gm output; ImageIn input; dx input; dy input; gd output; Ix output; Iy output
function [gm,gd,Ix,Iy]  = frameBasedMagTheta(ImageIn, dx, dy)
    [gm,gd,Ix,Iy] = hdl.npufun(@magThetaKernel, [3 3], ImageIn,'NonSampleInput',dx,'NonSampleInput',dy); 
end
 
function [gm,gd,Ix,Iy] = magThetaKernel(in,dx,dy) 
    dxTemp = in.*dx;
    Ix = sum(sum(dxTemp));

    dyTemp = in.*dy;
    Iy = sum(sum(dyTemp));

    gm = Ix.^2 + Iy.^2;   %Magnitude
    gd = atan2(Iy,Ix);    %Direction
end

== matlab function comboPlusKirschBinarized/combo/frameBasedGaussianFilter ==
  data: Result output; ImageIn input; data input
function Result   = frameBasedGaussianFilter(ImageIn, data)
    Result = hdl.npufun(@gaussianKernel, [3 3], ImageIn,'NonSampleInput', data); 
end
 
function e = gaussianKernel(in,data)
    temp = in.*data;
    e = sum(sum(temp));
end

== matlab function comboPlusKirschBinarized/combo/CocatTo64bits ==
  data: u1 input; y output; u2 input
function y = fcn(u1, u2)
% npu with a single element kernel 
y = hdl.npufun(@kernel, [1 1], u1, u2);

end

function out = kernel(in1, in2)
% use word2bits to get the bit representation of each input
a = hdl.word2bits(in1,32);
b = hdl.word2bits(in2,32);
% concatenate the bit vectors
out = bitconcat([a;b]);

end

== matlab function comboPlusKirschBinarized/combo/kirschFilterNorth/frameBasedKirschFilter ==
  data: Result output; ImageIn input; data input
function Result   = frameBasedKirschFilter(ImageIn, data)
    Result = hdl.npufun(@kirschKernel, [3 3], ImageIn,'NonSampleInput', data); 
end
 
function e = kirschKernel(in,data)
    temp = in.*data;
    e = abs(sum(sum(temp)));
end

== matlab function comboPlusKirschBinarized/combo/kirschFilterNorthWest/frameBasedKirschFilter ==
  data: Result output; ImageIn input; data input
function Result   = frameBasedKirschFilter(ImageIn, data)
    Result = hdl.npufun(@kirschKernel, [3 3], ImageIn,'NonSampleInput', data); 
end
 
function e = kirschKernel(in,data)
    temp = in.*data;
    e = abs(sum(sum(temp)));
end

== matlab function comboPlusKirschBinarized/combo/kirschFilterSouthWest/frameBasedKirschFilter ==
  data: Result output; ImageIn input; data input
function Result   = frameBasedKirschFilter(ImageIn, data)
    Result = hdl.npufun(@kirschKernel, [3 3], ImageIn,'NonSampleInput', data); 
end
 
function e = kirschKernel(in,data)
    temp = in.*data;
    e = abs(sum(sum(temp)));
end

== matlab function comboPlusKirschBinarized/combo/kirschFilterWest/frameBasedKirschFilter ==
  data: Result output; ImageIn input; data input
function Result   = frameBasedKirschFilter(ImageIn, data)
    Result = hdl.npufun(@kirschKernel, [3 3], ImageIn,'NonSampleInput', data); 
end
 
function e = kirschKernel(in,data)
    temp = in.*data;
    e = abs(sum(sum(temp)));
end

== matlab function comboPlusKirschBinarized/combo/statistics/frameBasedMean ==
  data: Result output; ImageIn input
function Result   = frameBasedMean(ImageIn)
    accumulator = single(0);    
    Result = hdl.iteratorfun(@max_fun, ImageIn, accumulator);
end
 
function accumulator = max_fun(sample, accumulator, idx)
  numPix = 40000;
  accumulator = accumulator + sample;
  if idx == numPix
    accumulator = single(accumulator / numPix);
  end
end

== matlab function comboPlusKirschBinarized/combo/statistics/frameBasedStd ==
  data: Result output; ImageIn input; mean input
function Result   = frameBasedStd(ImageIn, mean)
    accumulator2 = single(0);
    Result = hdl.iteratorfun(@max_fun2, ImageIn, accumulator2,mean); 
end
 
function accumulator2 = max_fun2(sample, accumulator2, idx, mean)
    numPix = 40000;  
    temp = (sample-mean)^2;
  accumulator2 = accumulator2 + temp;
  
  if idx == numPix
    accumulator2 = (accumulator2/(numPix - 1))^.5;
  end
end

== matlab function comboPlusKirschBinarized/combo/statistics1/frameBasedMean ==
  data: Result output; ImageIn input
function Result   = frameBasedMean(ImageIn)
    accumulator = single(0);    
    Result = hdl.iteratorfun(@max_fun, ImageIn, accumulator);
end
 
function accumulator = max_fun(sample, accumulator, idx)
  numPix = 40000;
  accumulator = accumulator + sample;
  if idx == numPix
    accumulator = single(accumulator / numPix);
  end
end
